simulink model "CenterLimit"  (R2016a)
settings: Solver=ode4  StartTime=0.0  StopTime=inf  FixedStep=ts  RelTol=1e-3
libraries: xpcmeasurementcomputinglib x7
settings Model: SimulationMode=external  Creator=Biorobotics  LastModifiedBy=Biorobotics
settings SolverCC: EnableConcurrentExecution=on
settings DataIOCC: SaveFormat=StructureWithTime
settings OptimizationCC: BlockReduction=off  OptimizeBlockIOStorage=off  BufferReuse=off  GlobalBufferReuse=off  ExpressionFolding=off  LocalBlockOutputs=off
settings HardwareCC: ProdBitPerPointer=32  ProdLargestAtomicFloat=None  ProdWordSize=32  ProdLongLongMode=on  ProdHWDeviceType=Generic->32-bit x86 compatible
settings RTWCC: SystemTargetFile=slrt.tlc  TemplateMakefile=slrt_default_tmf  Description=Simulink Real-Time  RTWCompilerOptimization=on

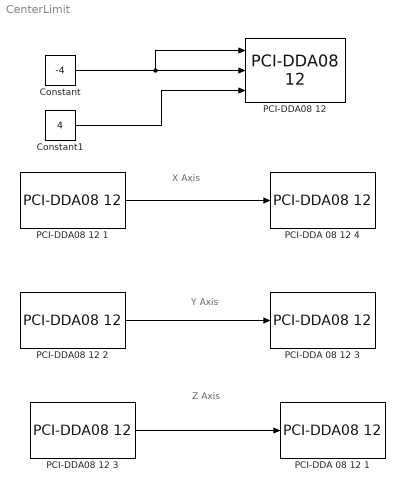
== system CenterLimit ==
  note: Y Axis
  note: Z Axis
  note: X Axis
  Constant : Constant  Value=-4
  Constant1 : Constant  Value=4
  PCI-DDA 08 12 1 : xpcmeasurementcomputinglib/Digital Output/PCI-DDA08 12   channel=5  port=A  reset=[1]  initValue=[0]  chip=1  sampletime=ts  slot=-1
  PCI-DDA 08 12 3 : xpcmeasurementcomputinglib/Digital Output/PCI-DDA08 12   channel=3  port=A  reset=[1]  initValue=[0]  chip=1  sampletime=ts  slot=-1
  PCI-DDA 08 12 4 : xpcmeasurementcomputinglib/Digital Output/PCI-DDA08 12   channel=1  port=A  reset=[1]  initValue=[0]  chip=1  sampletime=ts  slot=-1
  "PCI-DDA08 12 " : xpcmeasurementcomputinglib/D//A/PCI-DDA08 12   channel=[1 2 3]  range=[-10 -10 -10]  reset=[1]  initValue=[0]  sampletime=ts  pci_dev=-1
  PCI-DDA08 12 1 : xpcmeasurementcomputinglib/Digital Input/PCI-DDA08 12   channel=8  port=A  chip=2  sampletime=ts  slot=-1
  PCI-DDA08 12 2 : xpcmeasurementcomputinglib/Digital Input/PCI-DDA08 12   channel=8  port=B  chip=2  sampletime=ts  slot=-1
  PCI-DDA08 12 3 : xpcmeasurementcomputinglib/Digital Input/PCI-DDA08 12   channel=4  port=C  chip=2  sampletime=ts  slot=-1
  wires:
  Constant/1 -> "PCI-DDA08 12 "/2, "PCI-DDA08 12 "/1
  PCI-DDA08 12 1/1 -> PCI-DDA 08 12 4/1
  PCI-DDA08 12 2/1 -> PCI-DDA 08 12 3/1
  PCI-DDA08 12 3/1 -> PCI-DDA 08 12 1/1
  Constant1/1 -> "PCI-DDA08 12 "/3
